simulink model "cycloco"  (R2024b)
settings: Solver=VariableStepAuto  StartTime=0.0  StopTime=10.0  RelTol=1e-3
libraries: spsDetailedThyristorLib x4, spsVoltageMeasurementLib x2, spsACVoltageSourceLib x1, spsCurrentMeasurementLib x1, spsLinearTransformerLib x1, spsSeriesRLCBranchLib x1, sps_lib x1
settings Model: Creator=ETC  LastModifiedBy=ETC

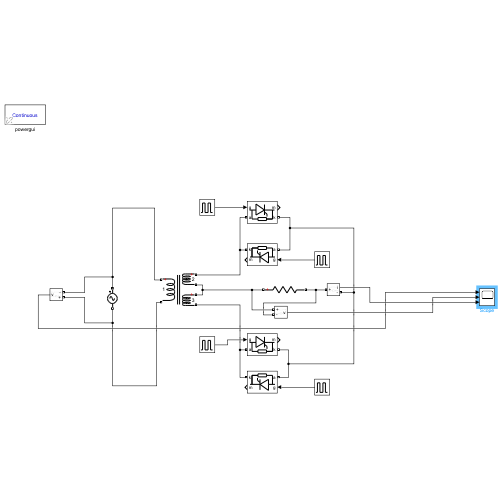
[thumbnail: Simulink's stored preview of the top-level diagram]
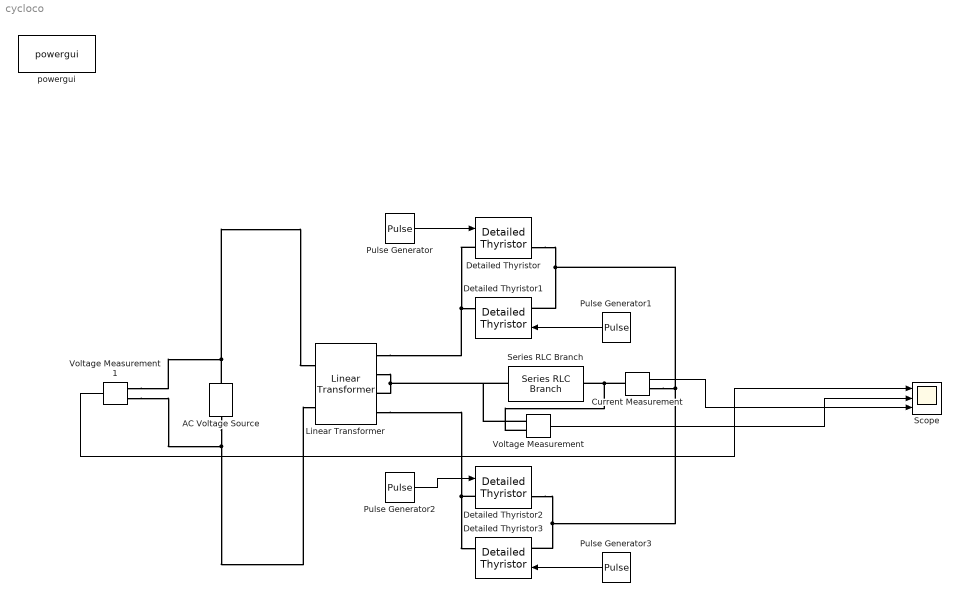
== system cycloco ==
  AC Voltage Source : spsACVoltageSourceLib/AC Voltage Source  Amplitude=10  Phase=0  Frequency=50  SampleTime=0  Measurements=None  BusType=swing  Pref=10e3  Qref=0  Qmin=-inf  Qmax=+inf
  Current Measurement : spsCurrentMeasurementLib/Current Measurement  PhasorSimulation=off  OutputType=Complex  PSBequivalent=0
  Detailed Thyristor{,1..3} (4 alike) : spsDetailedThyristorLib/Detailed Thyristor  Ron=0.001  Lon=1e-3  Vf=0.8  IL=0.1  Tq=100e-6  IC=0  Rs=500  Cs=250e-9  Measurements=on
      settings: LibrarySourceBlock=sps_lib/Power Electronics/Detailed Thyristor
  Linear Transformer : spsLinearTransformerLib/Linear Transformer  UNITS=pu  NominalPower=[ 250e6 60 ]  winding1="[ 735e3  0.002  0.08 ]"  winding2="[ 315e3  0.002  0.08 ]"  ThreeWindings=on  winding3=[ 315e3 0.002 0.08 ]  RmLm=[ 500 500 ]  Measurements=None  DataType=off
  Pulse Generator : DiscretePulseGenerator  PulseType=Time based  Period=0.08  PulseWidth=50
  Pulse Generator1 : DiscretePulseGenerator  PulseType=Time based  Period=0.08  PulseWidth=50
  Pulse Generator2 : DiscretePulseGenerator  PulseType=Time based  Period=0.08  PulseWidth=50  PhaseDelay=0.04
  Pulse Generator3 : DiscretePulseGenerator  PulseType=Time based  Period=0.08  PulseWidth=50  PhaseDelay=0.04
  Scope : Scope  NumInputPorts=3
  Series RLC Branch : spsSeriesRLCBranchLib/Series RLC Branch  LConnTagsString=__new0  RConnTagsString=__new0  BranchType=R  Resistance=100  Inductance=1e-3  SetiL0=off  InitialCurrent=0  Capacitance=1e-6  Setx0=off  InitialVoltage=0  Measurements=None
  Voltage Measurement : spsVoltageMeasurementLib/Voltage Measurement  PhasorSimulation=off  OutputType=Complex  PSBequivalent=0
  Voltage Measurement1 : spsVoltageMeasurementLib/Voltage Measurement  PhasorSimulation=off  OutputType=Complex  PSBequivalent=0
  powergui : sps_lib/powergui  Priority=1  SimulationMode=Continuous  SampleTime=50e-6  frequency=60  Iterations=50  frequencyindice=50  Pbase=100e6  ErrMax=1e-4  UnitsV=kV  UnitsW=MW  buscounter=0  FunctionMessages=off  echomessages=off  EnableUseOfTLC=off  CurrentSourceSwitches=off  DisableSnubberDevices=off  DisableRonSwitches=off  DisableVfSwitches=off  DisplayEquations=off  AutomaticDiscreteSolvers=off  SolverType=Tustin/Backward Euler (TBE)  Interpol=off  ExternalGateDelay=off  methode=off  Ts=100  x0status=blocks  SPID=on  SwTol=0  HookPort=off  NonlinearTolerance=1e-4  nMaxIteration=100  ContinueOnMaxIteration=off  RestoreLinks=warning  ResistiveCurrentMeasurement=off  Frange=[0:2:500]  Ylog=off  Xlog=on  ShowGrid=off  save=off  variable=ZData  structure=0  ZoomFFT=off  StartTime=0.0  cycles=1  DisplayStyle=1  fundamental=60  FreqAxis=off  MaxFrequency=1000  frequencyindicesteady=1  RmsSteady=1  display=off
  wires:
  Pulse Generator1/1 -> Detailed Thyristor1/1
  Pulse Generator/1 -> Detailed Thyristor/1
  Pulse Generator2/1 -> Detailed Thyristor2/1
  Pulse Generator3/1 -> Detailed Thyristor3/1
  Voltage Measurement1/1 -> Scope/1
  Voltage Measurement/1 -> Scope/2
  Current Measurement/1 -> Scope/3
  connections:
  Detailed Thyristor/LConn1 -- Linear Transformer/RConn1 -- Detailed Thyristor1/RConn1
  Detailed Thyristor2/LConn1 -- Detailed Thyristor3/RConn1 -- Linear Transformer/RConn4
  Linear Transformer/RConn2 -- Voltage Measurement/LConn1 -- Series RLC Branch/LConn1 -- Linear Transformer/RConn3
  Current Measurement/LConn1 -- Voltage Measurement/LConn2 -- Series RLC Branch/RConn1
  Detailed Thyristor2/RConn1 -- Current Measurement/RConn1 -- Detailed Thyristor1/LConn1 -- Detailed Thyristor/RConn1 -- Detailed Thyristor3/LConn1
  AC Voltage Source/RConn1 -- Linear Transformer/LConn1 -- Voltage Measurement1/LConn2
  AC Voltage Source/LConn1 -- Linear Transformer/LConn2 -- Voltage Measurement1/LConn1
